simulink model "kalman_sim"  (R2017b)
settings: Solver=ode4  StartTime=0.0  StopTime=2000  FixedStep=5  RelTol=1e-3
values from neighbouring files (symbols this model uses):
  A = [-.0213 0 0; 0.0006 -0.005 0;0 -0.00038 -0.0023]    [kalman.m]    (also in med.m = [A11 A12 ; A21 A22]; oneforall.m = [A11 A12 ; A21 A22]; oneinall_utf8.m = [A11 A12 ; A21 A22])
  B = [8.9362;0;0]    [kalman.m]    (also in med.m = [0;1/m]; oneforall.m = [0;1/m]; oneinall_utf8.m = [0;1/m])
  C = eye(3)    [kalman.m]    (also in med.m = [1 0]; oneforall.m = [1 0]; oneinall_utf8.m = [1 0])
  K = place(A,B,P)    [oneforall.m]    (also in oneinall_utf8.m)
  M = [0.1 0 0;0 0.1 0;0 0 0.00132]    [kalman.m]    (also in oneforall.m = [0.1 0 0 0; 0 0.1 0 0; 0 0 0.00132 0 ;0 0 0 0.1]; oneinall_utf8.m = [0.1 0 0 0; 0 0.1 0 0; 0 0 0.00132 0 ;0 0 0 0.1])
settings Model: Creator=lencs  LastModifiedBy=lencs

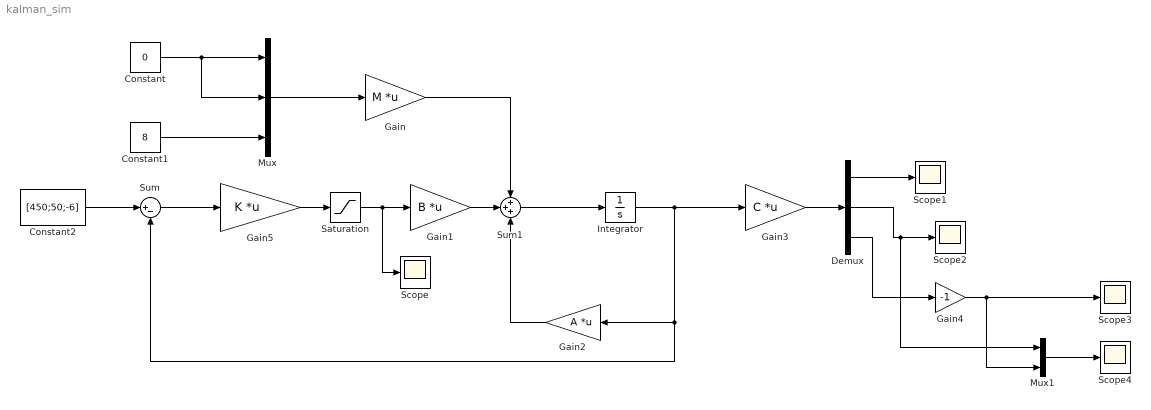
== system kalman_sim ==
  Constant : Constant  Value=0
  Constant1 : Constant  Value=8
  Constant2 : Constant  Value=[450;50;-6]
  Demux : Demux  Outputs=3
  Gain : Gain  Gain=M  Multiplication=Matrix(K*u) (u vector)
  Gain1 : Gain  Gain=B  Multiplication=Matrix(K*u) (u vector)
  Gain2 : Gain  Gain=A  Multiplication=Matrix(K*u)
  Gain3 : Gain  Gain=C  Multiplication=Matrix(K*u) (u vector)
  Gain4 : Gain  Gain=-1
  Gain5 : Gain  Gain=K  Multiplication=Matrix(K*u) (u vector)
  Integrator : Integrator  InitialCondition=[200; 30; -30]
  Mux : Mux  Inputs=3
  Mux1 : Mux  Inputs=2
  Saturation : Saturate  UpperLimit=pi/2  LowerLimit=0
  Scope{,1..4} (5 alike) : Scope
  Sum : Sum  Inputs=|+-
  Sum1 : Sum  Inputs=+++
  wires:
  Constant/1 -> Mux/2, Mux/1
  Constant1/1 -> Mux/3
  Mux/1 -> Gain/1
  Constant2/1 -> Sum/1
  Saturation/1 -> Scope/1, Gain1/1
  Gain1/1 -> Sum1/2
  Gain/1 -> Sum1/1
  Sum1/1 -> Integrator/1
  Integrator/1 -> Sum/2, Gain2/1, Gain3/1
  Gain3/1 -> Demux/1
  Demux/1 -> Scope1/1
  Demux/2 -> Mux1/1, Scope2/1
  Gain2/1 -> Sum1/3
  Sum/1 -> Gain5/1
  Gain5/1 -> Saturation/1
  Demux/3 -> Gain4/1
  Gain4/1 -> Mux1/2, Scope3/1
  Mux1/1 -> Scope4/1
